simulink library "LinkedSubsytems"  (R2023a)
settings: Solver=VariableStepAuto  StartTime=0.0  StopTime=10.0  RelTol=1e-3
settings Model: Creator=Tre'Vaughn  LastModifiedBy=Tre'Vaughn

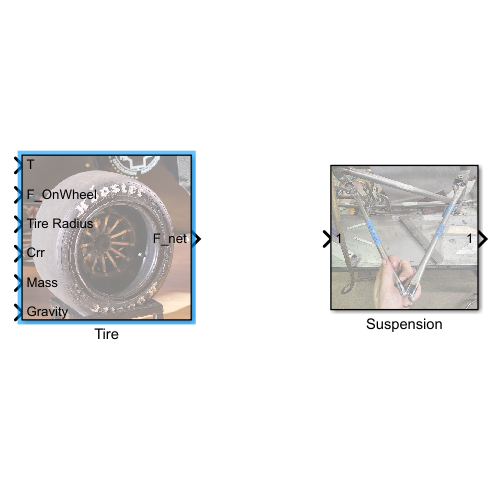
[thumbnail: Simulink's stored preview of the top-level diagram]
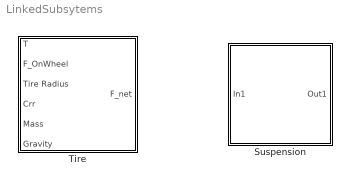
== system LinkedSubsytems ==
  Suspension : Subsystem
      mask Display: image('C:\Users\Tre''Vaughn\Documents\MATLAB\RMSimModel\Subsystem Pics\Suspension.jpg'); % Use "Edit Image" on toolstrip to change.
  Tire : Subsystem
      mask Display: image('C:\Users\Tre''Vaughn\Documents\MATLAB\RMSimModel\Subsystem Pics\TIre 50.png'); % Use "Edit Image" on toolstrip to change.

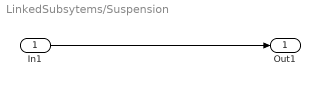
== system LinkedSubsytems/Suspension ==
  In1 : Inport
  Out1 : Outport
  wires:
  In1/1 -> Out1/1

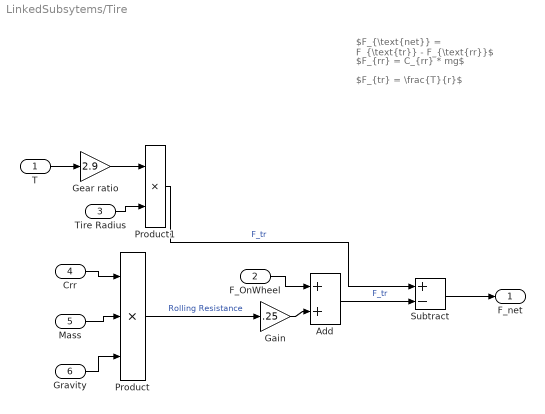
== system LinkedSubsytems/Tire ==
  note: $F_{tr} = \frac{T}{r}$
  note: $F_{\text{net}} = F_{\text{tr}} - F_{\text{rr}}$
  note: $F_{rr} = C_{rr} * mg$
  T : Inport
  F_OnWheel : Inport  Port=2
  Tire Radius : Inport  Port=3
  Crr : Inport  Port=4
  Mass : Inport  Port=5
  Gravity : Inport  Port=6
  Add : Sum
  Gain : Gain  Gain=.25
  Gear ratio : Gain  Gain=2.9
  Product : Product  Inputs=3
  Product1 : Product
  Subtract : Sum  Inputs=+-
  F_net : Outport
  wires:
  Mass/1 -> Product/2
  Crr/1 -> Product/1
  Gravity/1 -> Product/3
  Product/1 -> Gain/1  "Rolling Resistance"
  T/1 -> Gear ratio/1
  Tire Radius/1 -> Product1/2
  F_OnWheel/1 -> Add/1
  Add/1 -> Subtract/2  "F_tr"
  Product1/1 -> Subtract/1  "F_tr"
  Subtract/1 -> F_net/1
  Gain/1 -> Add/2
  Gear ratio/1 -> Product1/1
